simulink model "SV16"  (R2026a)
settings: Solver=VariableStepAuto  StopTime=0.1
libraries: simulink x55, hdlsllib x34
(part 1 of 2)
settings Model: Creator=Soham  LastModifiedBy=Soham

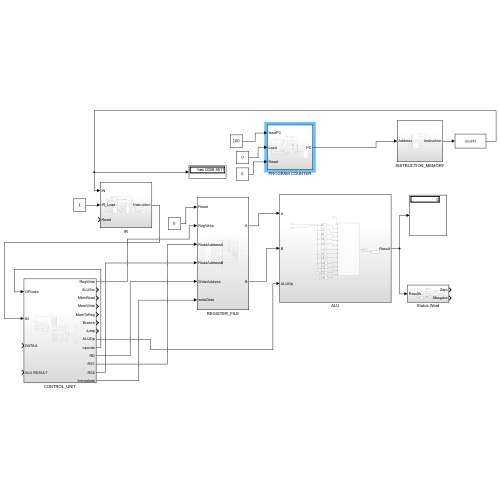
[thumbnail: Simulink's stored preview of the top-level diagram]
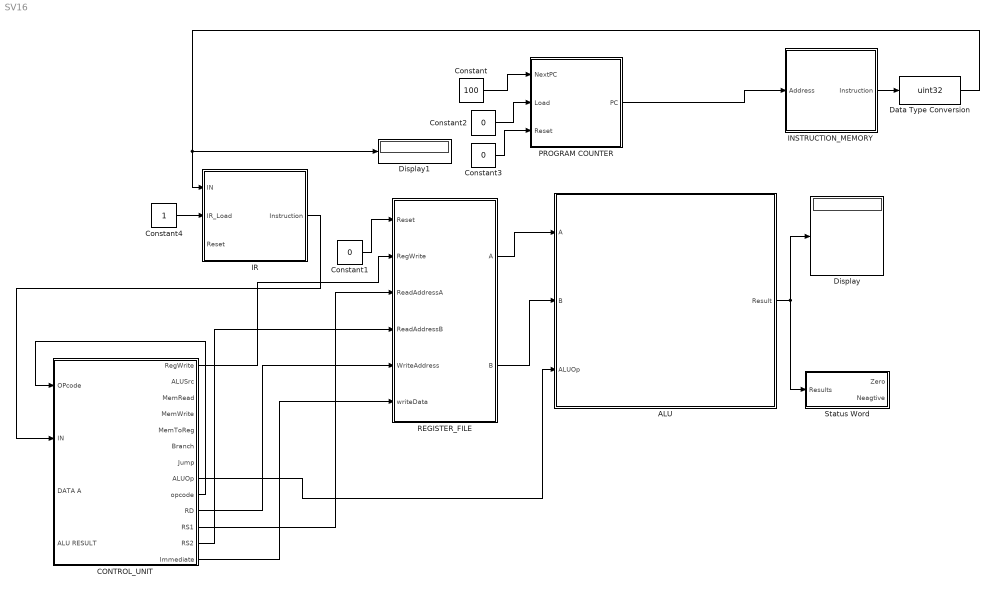
== system SV16 ==
  ALU : Subsystem
  CONTROL_UNIT : Subsystem
  Constant : Constant  Value=100  OutDataTypeStr=uint32
  Constant1 : Constant  Value=0  OutDataTypeStr=uint16
  Constant2 : Constant  Value=0  OutDataTypeStr=uint32
  Constant3 : Constant  Value=0
  Constant4 : Constant  OutDataTypeStr=uint32
  Data Type Conversion : DataTypeConversion  OutDataTypeStr=uint32  SaturateOnIntegerOverflow=off  RndMeth=Floor
  Display : Display
  Display1 : Display
      settings: Format=hex (Stored Integer)
  INSTRUCTION_MEMORY : Subsystem
  IR : Subsystem
  PROGRAM COUNTER : Subsystem
  REGISTER_FILE : Subsystem
  Status Word : Subsystem
  wires:
  Constant1/1 -> REGISTER_FILE/1(Reset)
  REGISTER_FILE/1(A) -> ALU/1(A)
  REGISTER_FILE/2(B) -> ALU/2(B)
  ALU/1(Result) -> Display/1, Status Word/1(Results)
  CONTROL_UNIT/8(ALUOp) -> ALU/3(ALUOp)
  CONTROL_UNIT/1(RegWrite) -> REGISTER_FILE/2(RegWrite)
  Data Type Conversion/1 -> IR/1(IN), Display1/1
  Constant4/1 -> IR/2(IR_Load)
  IR/1(Instruction) -> CONTROL_UNIT/2(IN)
  CONTROL_UNIT/11(RS1) -> REGISTER_FILE/3(ReadAddressA)
  CONTROL_UNIT/12(RS2) -> REGISTER_FILE/4(ReadAddressB)
  CONTROL_UNIT/10(RD) -> REGISTER_FILE/5(WriteAddress)
  CONTROL_UNIT/13(Immediate) -> REGISTER_FILE/6(writeData)
  CONTROL_UNIT/9(opcode) -> CONTROL_UNIT/1(OPcode)
  INSTRUCTION_MEMORY/1(Instruction) -> Data Type Conversion/1
  PROGRAM COUNTER/1(PC) -> INSTRUCTION_MEMORY/1(Address)
  Constant/1 -> PROGRAM COUNTER/1(NextPC)
  Constant2/1 -> PROGRAM COUNTER/2(Load)
  Constant3/1 -> PROGRAM COUNTER/3(Reset)

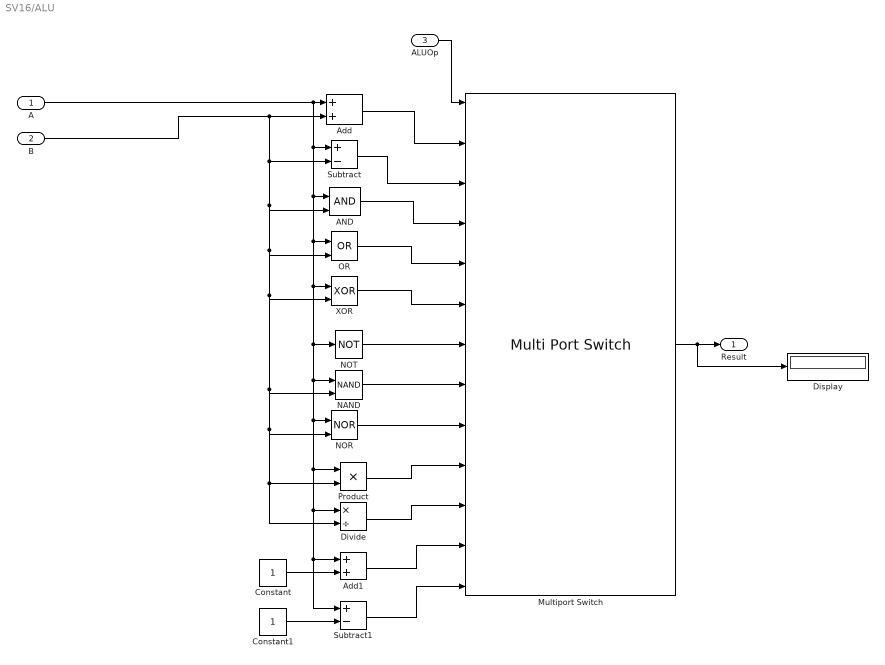
== system SV16/ALU ==
  A : Inport  OutDataTypeStr=uint16
  B : Inport  Port=2  OutDataTypeStr=uint16
  ALUOp : Inport  Port=3  OutDataTypeStr=uint8
  AND : Logic  IconShape=distinctive  AllPortsSameDT=off  OutDataTypeStr=boolean
  Add : Sum
  Add1 : Sum
  Constant : Constant  OutDataTypeStr=uint16
  Constant1 : Constant  OutDataTypeStr=uint16
  Display : Display
  Divide : Product  Inputs=*/
  Multiport Switch : MultiPortSwitch  DataPortOrder=Zero-based contiguous  Inputs=12  zeroidx=on  OutDataTypeStr=uint16  SaturateOnIntegerOverflow=off  InputSameDT=off
  NAND : Logic  Operator=NAND  IconShape=distinctive  AllPortsSameDT=off  OutDataTypeStr=boolean
  NOR : Logic  Operator=NOR  IconShape=distinctive  AllPortsSameDT=off  OutDataTypeStr=boolean
  NOT : Logic  Operator=NOT  IconShape=distinctive  AllPortsSameDT=off  OutDataTypeStr=boolean
  OR : Logic  Operator=OR  IconShape=distinctive  AllPortsSameDT=off  OutDataTypeStr=boolean
  Product : Product
  Subtract : Sum  Inputs=+-
  Subtract1 : Sum  Inputs=+-
  XOR : Logic  Operator=XOR  IconShape=distinctive  AllPortsSameDT=off  OutDataTypeStr=boolean
  Result : Outport  OutDataTypeStr=uint16
  wires:
  Constant/1 -> Add1/2
  Constant1/1 -> Subtract1/2
  ALUOp/1 -> Multiport Switch/1
  Multiport Switch/1 -> Display/1, Result/1
  A/1 -> AND/1, Subtract1/1, Add1/1, Divide/1, Product/1, NOR/1, NAND/1, NOT/1, XOR/1, OR/1, Subtract/1, Add/1
  Add/1 -> Multiport Switch/2
  Subtract/1 -> Multiport Switch/3
  AND/1 -> Multiport Switch/4
  OR/1 -> Multiport Switch/5
  XOR/1 -> Multiport Switch/6
  NOT/1 -> Multiport Switch/7
  NAND/1 -> Multiport Switch/8
  NOR/1 -> Multiport Switch/9
  Subtract1/1 -> Multiport Switch/13
  Add1/1 -> Multiport Switch/12
  Divide/1 -> Multiport Switch/11
  Product/1 -> Multiport Switch/10
  B/1 -> NAND/2, Divide/2, Product/2, NOR/2, XOR/2, OR/2, AND/2, Subtract/2, Add/2

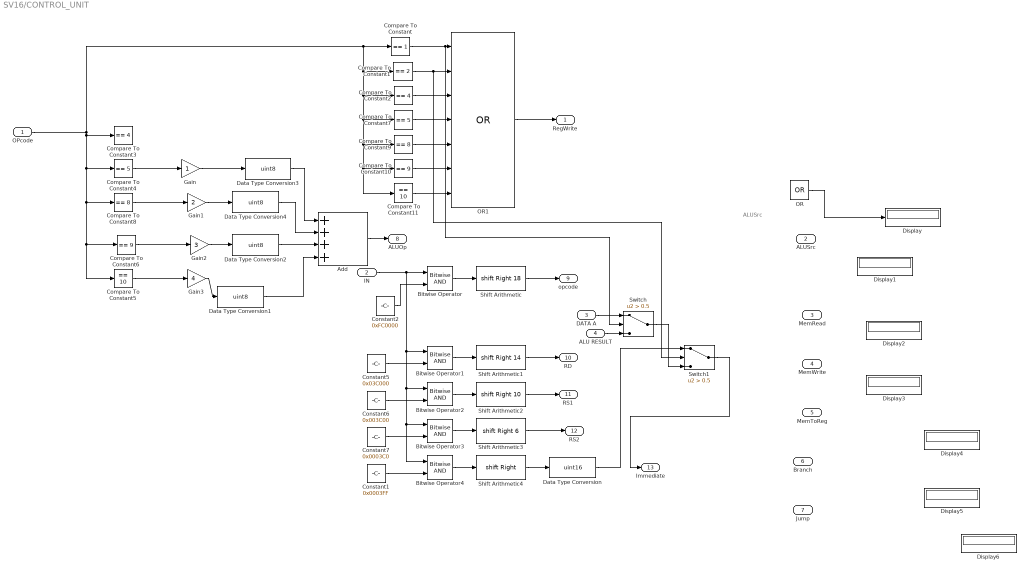
== system SV16/CONTROL_UNIT ==
  note: ALUSrc
  OPcode : Inport  OutDataTypeStr=uint32  PortDimensions=1
  IN : Inport  Port=2
  DATA A : Inport  Port=3
  ALU RESULT : Inport  Port=4
  Add : Sum  Inputs=++++
  Bitwise Operator{,1..4} (5 alike) : simulink/Logic and Bit Operations/Bitwise Operator  logicop=AND  UseBitMask=off  NumInputPorts=2  BitMask=bin2dec('11011001')  BitMaskRealWorld=Stored Integer
  Compare To Constant : simulink/Logic and Bit Operations/Compare To Constant  relop===  const=1  OutDataTypeStr=boolean
  Compare To Constant1 : simulink/Logic and Bit Operations/Compare To Constant  relop===  const=2  OutDataTypeStr=boolean
  Compare To Constant10 : simulink/Logic and Bit Operations/Compare To Constant  relop===  const=9  OutDataTypeStr=boolean
  Compare To Constant11 : simulink/Logic and Bit Operations/Compare To Constant  relop===  const=10  OutDataTypeStr=boolean
  Compare To Constant2 : simulink/Logic and Bit Operations/Compare To Constant  relop===  const=4  OutDataTypeStr=boolean
  Compare To Constant3 : simulink/Logic and Bit Operations/Compare To Constant  relop===  const=4  OutDataTypeStr=boolean
  Compare To Constant4 : simulink/Logic and Bit Operations/Compare To Constant  relop===  const=5  OutDataTypeStr=boolean
  Compare To Constant5 : simulink/Logic and Bit Operations/Compare To Constant  relop===  const=10  OutDataTypeStr=boolean
  Compare To Constant6 : simulink/Logic and Bit Operations/Compare To Constant  relop===  const=9  OutDataTypeStr=boolean
  Compare To Constant7 : simulink/Logic and Bit Operations/Compare To Constant  relop===  const=5  OutDataTypeStr=boolean
  Compare To Constant8 : simulink/Logic and Bit Operations/Compare To Constant  relop===  const=8  OutDataTypeStr=boolean
  Compare To Constant9 : simulink/Logic and Bit Operations/Compare To Constant  relop===  const=8  OutDataTypeStr=boolean
  Constant1 : Constant  Value=0x0003FF
  Constant2 : Constant  Value=0xFC0000
  Constant5 : Constant  Value=0x03C000
  Constant6 : Constant  Value=0x003C00
  Constant7 : Constant  Value=0x0003C0
  Data Type Conversion : DataTypeConversion  OutDataTypeStr=uint16  SaturateOnIntegerOverflow=off  RndMeth=Floor
  Data Type Conversion{1..4} (4 alike) : DataTypeConversion  OutDataTypeStr=uint8  SaturateOnIntegerOverflow=off  RndMeth=Floor
  Display{,1..6} (7 alike) : Display
  Gain : Gain
  Gain1 : Gain  Gain=2
  Gain2 : Gain  Gain=3
  Gain3 : Gain  Gain=4
  OR : Logic  Operator=OR  IconShape=distinctive  AllPortsSameDT=off  OutDataTypeStr=boolean
  OR1 : Logic  Operator=OR  Inputs=7  IconShape=distinctive  AllPortsSameDT=off  OutDataTypeStr=boolean
  Shift Arithmetic : ArithShift  BitShiftNumber=18  BitShiftDirection=Right
  Shift Arithmetic1 : ArithShift  BitShiftNumber=14  BitShiftDirection=Right
  Shift Arithmetic2 : ArithShift  BitShiftNumber=10  BitShiftDirection=Right
  Shift Arithmetic3 : ArithShift  BitShiftNumber=6  BitShiftDirection=Right
  Shift Arithmetic4 : ArithShift  BitShiftDirection=Right
  Switch : Switch  Criteria=u2 > Threshold  Threshold=0.5  SaturateOnIntegerOverflow=off  InputSameDT=off
  Switch1 : Switch  Criteria=u2 > Threshold  Threshold=0.5  SaturateOnIntegerOverflow=off  InputSameDT=off
  RegWrite : Outport  OutDataTypeStr=boolean
  ALUSrc : Outport  Port=2  OutDataTypeStr=boolean
  MemRead : Outport  Port=3  OutDataTypeStr=boolean
  MemWrite : Outport  Port=4  OutDataTypeStr=boolean
  MemToReg : Outport  Port=5  OutDataTypeStr=boolean
  Branch : Outport  Port=6  OutDataTypeStr=boolean
  Jump : Outport  Port=7  OutDataTypeStr=boolean
  ALUOp : Outport  Port=8  OutDataTypeStr=uint8
  opcode : Outport  Port=9
  RD : Outport  Port=10
  RS1 : Outport  Port=11
  RS2 : Outport  Port=12
  Immediate : Outport  Port=13
  wires:
  ? -> OR/1
  ? -> OR/2
  OR/1 -> Display/1
  ? -> Display1/1, ALUSrc/1
  ? -> Display2/1, MemRead/1
  ? -> Display3/1, MemWrite/1
  ? -> Display4/1, MemToReg/1
  ? -> Display5/1, Branch/1
  ? -> Display6/1, Jump/1
  OPcode/1 -> Compare To Constant11/1, Compare To Constant10/1, Compare To Constant9/1, Compare To Constant7/1, Compare To Constant2/1, Compare To Constant1/1, Compare To Constant/1, Compare To Constant4/1, Compare To Constant5/1, Compare To Constant6/1, Compare To Constant8/1, Compare To Constant3/1
  Compare To Constant/1 -> OR1/1, Switch/2
  Compare To Constant8/1 -> Gain1/1
  Compare To Constant4/1 -> Gain/1
  Compare To Constant6/1 -> Gain2/1
  Compare To Constant5/1 -> Gain3/1
  Compare To Constant1/1 -> Switch1/2, OR1/2
  Gain/1 -> Data Type Conversion3/1
  Gain2/1 -> Data Type Conversion2/1
  Gain1/1 -> Data Type Conversion4/1
  Gain3/1 -> Data Type Conversion1/1
  Add/1 -> ALUOp/1
  Compare To Constant2/1 -> OR1/3
  Compare To Constant7/1 -> OR1/4
  Compare To Constant9/1 -> OR1/5
  Compare To Constant10/1 -> OR1/6
  Compare To Constant11/1 -> OR1/7
  OR1/1 -> RegWrite/1
  Bitwise Operator3/1 -> Shift Arithmetic3/1
  Constant7/1 -> Bitwise Operator3/2
  Bitwise Operator2/1 -> Shift Arithmetic2/1
  Constant2/1 -> Bitwise Operator/2
  Bitwise Operator/1 -> Shift Arithmetic/1
  Constant5/1 -> Bitwise Operator1/2
  Bitwise Operator1/1 -> Shift Arithmetic1/1
  Constant1/1 -> Bitwise Operator4/2
  Shift Arithmetic1/1 -> RD/1
  Shift Arithmetic3/1 -> RS2/1
  Constant6/1 -> Bitwise Operator2/2
  Bitwise Operator4/1 -> Shift Arithmetic4/1
  Shift Arithmetic4/1 -> Data Type Conversion/1
  Shift Arithmetic/1 -> opcode/1
  Shift Arithmetic2/1 -> RS1/1
  IN/1 -> Bitwise Operator4/1, Bitwise Operator3/1, Bitwise Operator2/1, Bitwise Operator1/1, Bitwise Operator/1
  DATA A/1 -> Switch/1
  ALU RESULT/1 -> Switch/3
  Switch/1 -> Switch1/3
  Data Type Conversion/1 -> Switch1/1
  Switch1/1 -> Immediate/1
  Data Type Conversion1/1 -> Add/4
  Data Type Conversion2/1 -> Add/3
  Data Type Conversion3/1 -> Add/1
  Data Type Conversion4/1 -> Add/2

== system SV16/INSTRUCTION_MEMORY ==
  Address : Inport  OutDataTypeStr=uint32
  Compare To Constant : simulink/Logic and Bit Operations/Compare To Constant  relop=>=  const=8  OutDataTypeStr=boolean
  Constant : Constant  Value=0x088011  VectorParams1D=off
  Constant1 : Constant  OutDataTypeStr=boolean
  Constant2 : Constant  Value=0x088011  VectorParams1D=off
  Data Type Conversion : DataTypeConversion  OutDataTypeStr=uint32  SaturateOnIntegerOverflow=off  RndMeth=Floor
  Display : Display
      settings: Format=hex (Stored Integer)
  Display1 : Display
      settings: Format=hex (Stored Integer)
  Display2 : Display
      settings: Format=hex (Stored Integer)
  MEMORY_BANK_8_B0 : Subsystem
  MEMORY_BANK_8_B1 : Subsystem
  Subsystem : Subsystem
  Switch : Switch  Criteria=u2 ~= 0  SaturateOnIntegerOverflow=off  InputSameDT=off
  Instruction : Outport  OutDataTypeStr=uint32
  wires:
  MEMORY_BANK_8_B0/1(DataOut) -> Switch/3, Display/1
  Address/1 -> Subsystem/1(IN)
  Subsystem/1(AD0) -> MEMORY_BANK_8_B0/2(Address0)
  Subsystem/2(AD1) -> MEMORY_BANK_8_B0/3(Address1)
  Subsystem/3(AD2) -> MEMORY_BANK_8_B0/4(Address2)
  Subsystem/4(INSTRUCTION INDEX) -> Compare To Constant/1
  Compare To Constant/1 -> Switch/2
  MEMORY_BANK_8_B1/1(DataOut) -> Switch/1, Display1/1
  Switch/1 -> Display2/1, Data Type Conversion/1
  Data Type Conversion/1 -> Instruction/1
  Constant/1 -> MEMORY_BANK_8_B0/1(DataIn)
  Constant1/1 -> MEMORY_BANK_8_B0/6(WriteEnable), MEMORY_BANK_8_B1/6(WriteEnable)
  Constant2/1 -> MEMORY_BANK_8_B1/1(DataIn)

== system SV16/IR ==
  IN : Inport  OutDataTypeStr=uint32
  IR_Load : Inport  Port=2  OutDataTypeStr=uint32
  Reset : Inport  Port=3  OutDataTypeStr=uint32
  Constant : Constant  Value=0  OutDataTypeStr=uint32
  Constant1 : Constant  OutDataTypeStr=uint32
  Display : Display
  Switch : Switch  Criteria=u2 > Threshold  SaturateOnIntegerOverflow=off  InputSameDT=off
  Switch1 : Switch  Criteria=u2 > Threshold  OutDataTypeStr=uint32  SaturateOnIntegerOverflow=off  InputSameDT=off
  Unit Delay Enabled Synchronous : hdlsllib/Discrete/Unit Delay Enabled Synchronous  InitialCondition=0.0  SampleTime=-1
  Instruction : Outport  OutDataTypeStr=uint32  PortDimensions=1
  wires:
  IN/1 -> Switch/1
  IR_Load/1 -> Switch/2
  Reset/1 -> Switch1/2
  Constant/1 -> Switch1/1
  Switch/1 -> Switch1/3
  Unit Delay Enabled Synchronous/1 -> Switch/3, Display/1, Instruction/1
  Switch1/1 -> Unit Delay Enabled Synchronous/1
  Constant1/1 -> Unit Delay Enabled Synchronous/2

== system SV16/PROGRAM COUNTER ==
  NextPC : Inport  OutDataTypeStr=uint32
  Load : Inport  Port=2  OutDataTypeStr=uint32
  Reset : Inport  Port=3
  Add : Sum
  Constant1 : Constant
  Constant2 : Constant  Value=3
  Constant3 : Constant  Value=0
  Data Type Conversion : DataTypeConversion  OutDataTypeStr=uint32  SaturateOnIntegerOverflow=off  RndMeth=Floor
  Data Type Conversion1 : DataTypeConversion  OutDataTypeStr=uint32  SaturateOnIntegerOverflow=off  RndMeth=Floor
  Display : Display
      settings: Format=decimal (Stored Integer)
  Unit Delay Enabled Synchronous : hdlsllib/Discrete/Unit Delay Enabled Synchronous  InitialCondition=0.0  SampleTime=0.001
  pc switch : Switch  Criteria=u2 > Threshold  OutDataTypeStr=uint32  SaturateOnIntegerOverflow=off  InputSameDT=off
  reset switch : Switch  Criteria=u2 > Threshold  SaturateOnIntegerOverflow=off  InputSameDT=off
  PC : Outport  OutDataTypeStr=uint32
  wires:
  Constant1/1 -> Unit Delay Enabled Synchronous/2
  Unit Delay Enabled Synchronous/1 -> Add/2, PC/1, Display/1
  Constant2/1 -> Add/1
  NextPC/1 -> pc switch/1
  Load/1 -> pc switch/2
  Add/1 -> pc switch/3
  Constant3/1 -> reset switch/1
  Reset/1 -> reset switch/2
  pc switch/1 -> Data Type Conversion1/1
  reset switch/1 -> Data Type Conversion/1
  Data Type Conversion/1 -> Unit Delay Enabled Synchronous/1
  Data Type Conversion1/1 -> reset switch/3

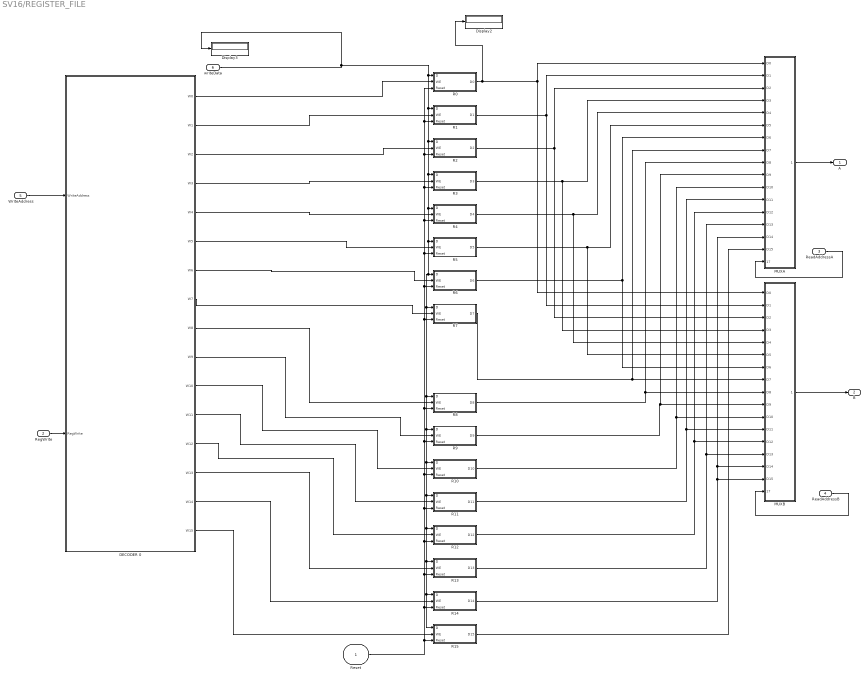
== system SV16/REGISTER_FILE ==
  Reset : Inport
  RegWrite : Inport  Port=2
  ReadAddressA : Inport  Port=3
  ReadAddressB : Inport  Port=4
  WriteAddress : Inport  Port=5
  writeData : Inport  Port=6
  DECODER 0 : Subsystem
  Display2 : Display
  Display3 : Display
  MUXA : Subsystem
  MUXB : Subsystem
  R0 : Subsystem
  R1 : Subsystem
  R10 : Subsystem
  R11 : Subsystem
  R12 : Subsystem
  R13 : Subsystem
  R14 : Subsystem
  R15 : Subsystem
  R2 : Subsystem
  R3 : Subsystem
  R4 : Subsystem
  R5 : Subsystem
  R6 : Subsystem
  R7 : Subsystem
  R8 : Subsystem
  R9 : Subsystem
  A : Outport  OutDataTypeStr=uint16
  B : Outport  Port=2  OutDataTypeStr=uint16
  wires:
  DECODER 0/1(W0) -> R0/2(WE)
  DECODER 0/2(W1) -> R1/2(WE)
  DECODER 0/3(W2) -> R2/2(WE)
  DECODER 0/4(W3) -> R3/2(WE)
  DECODER 0/5(W4) -> R4/2(WE)
  DECODER 0/6(W5) -> R5/2(WE)
  DECODER 0/7(W6) -> R6/2(WE)
  DECODER 0/8(W7) -> R7/2(WE)
  R0/1(D0) -> Display2/1, MUXA/1(D0), MUXB/1(D0)
  R1/1(D1) -> MUXA/2(D1), MUXB/2(D1)
  R2/1(D2) -> MUXB/3(D2), MUXA/3(D2)
  R3/1(D3) -> MUXA/4(D3), MUXB/4(D3)
  R4/1(D4) -> MUXB/5(D4), MUXA/5(D4)
  R5/1(D5) -> MUXB/6(D5), MUXA/6(D5)
  R6/1(D6) -> MUXB/7(D6), MUXA/7(D6)
  R7/1(D7) -> MUXA/8(D7), MUXB/8(D7)
  writeData/1 -> R1/1(D), R2/1(D), R3/1(D), R4/1(D), R5/1(D), R15/1(D), R14/1(D), R13/1(D), R12/1(D), R11/1(D), R10/1(D), R9/1(D), R8/1(D), R7/1(D), R6/1(D), R0/1(D), Display3/1
  Reset/1 -> R13/3(Reset), R12/3(Reset), R11/3(Reset), R9/3(Reset), R8/3(Reset), R7/3(Reset), R6/3(Reset), R5/3(Reset), R4/3(Reset), R3/3(Reset), R2/3(Reset), R1/3(Reset), R0/3(Reset), R10/3(Reset), R14/3(Reset), R15/3(Reset)
  WriteAddress/1 -> DECODER 0/1(WriteAddress)
  RegWrite/1 -> DECODER 0/2(RegWrite)
  MUXA/1(ReadDataA) -> A/1
  MUXB/1(ReadDataB) -> B/1
  ReadAddressA/1 -> MUXA/17(ReadAddressA)
  ReadAddressB/1 -> MUXB/17(ReadAddressB)
  DECODER 0/9(W8) -> R8/2(WE)
  DECODER 0/10(W9) -> R9/2(WE)
  DECODER 0/11(W10) -> R10/2(WE)
  DECODER 0/12(W11) -> R11/2(WE)
  DECODER 0/13(W12) -> R12/2(WE)
  DECODER 0/14(W13) -> R13/2(WE)
  DECODER 0/15(W14) -> R14/2(WE)
  DECODER 0/16(W15) -> R15/2(WE)
  R8/1(D8) -> MUXA/9(D8), MUXB/9(D8)
  R9/1(D9) -> MUXA/10(D9), MUXB/10(D9)
  R10/1(D10) -> MUXA/11(D10), MUXB/11(D10)
  R11/1(D11) -> MUXA/12(D11), MUXB/12(D11)
  R12/1(D12) -> MUXA/13(D12), MUXB/13(D12)
  R13/1(D13) -> MUXA/14(D13), MUXB/14(D13)
  R14/1(D14) -> MUXA/15(D14), MUXB/15(D14), MUXB/16(D15)
  R15/1(D15) -> MUXA/16(D15)

== system SV16/Status Word ==
  Results : Inport  OutDataTypeStr=uint16
  Compare To Constant : simulink/Logic and Bit Operations/Compare To Constant  relop===  const=0  OutDataTypeStr=boolean
  Compare To Constant1 : simulink/Logic and Bit Operations/Compare To Constant  relop=>=  const=32768  OutDataTypeStr=boolean
  Display : Display
  Display1 : Display
  Zero : Outport  OutDataTypeStr=boolean
  Neagtive : Outport  Port=2
  wires:
  Results/1 -> Compare To Constant/1, Compare To Constant1/1
  Compare To Constant/1 -> Display/1, Zero/1
  Compare To Constant1/1 -> Display1/1, Neagtive/1

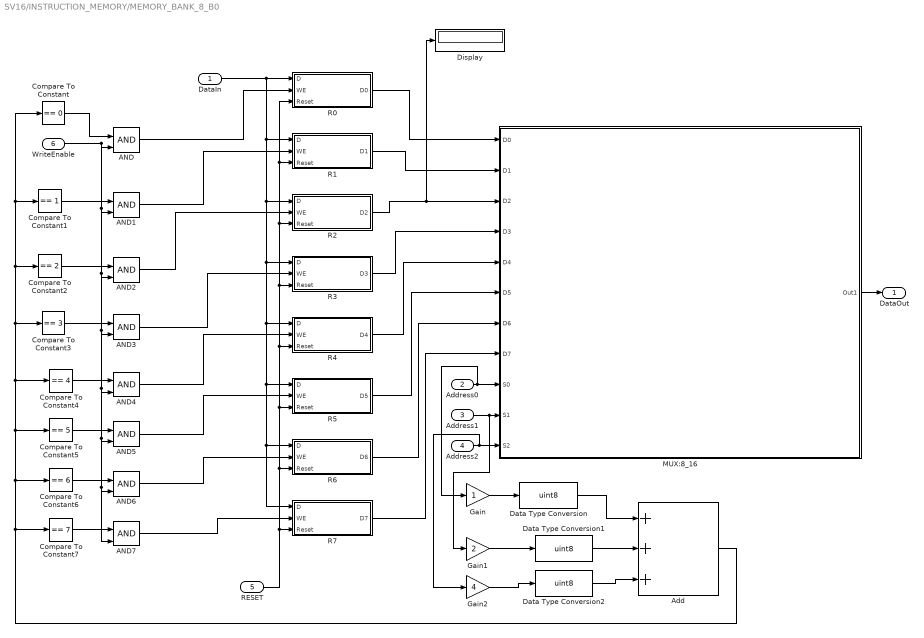
== system SV16/INSTRUCTION_MEMORY/MEMORY_BANK_8_B0 ==
  DataIn : Inport  OutDataTypeStr=uint32
  Address0 : Inport  Port=2  OutDataTypeStr=boolean
  Address1 : Inport  Port=3  OutDataTypeStr=boolean
  Address2 : Inport  Port=4  OutDataTypeStr=boolean
  RESET : Inport  Port=5  OutDataTypeStr=boolean
  WriteEnable : Inport  Port=6  OutDataTypeStr=boolean
  AND{,1..7} (8 alike) : Logic  IconShape=distinctive  AllPortsSameDT=off  OutDataTypeStr=boolean
  Add : Sum  Inputs=+++  OutDataTypeStr=Inherit: Inherit via back propagation
  Compare To Constant : simulink/Logic and Bit Operations/Compare To Constant  relop===  const=0  OutDataTypeStr=boolean
  Compare To Constant1 : simulink/Logic and Bit Operations/Compare To Constant  relop===  const=1  OutDataTypeStr=boolean
  Compare To Constant2 : simulink/Logic and Bit Operations/Compare To Constant  relop===  const=2  OutDataTypeStr=boolean
  Compare To Constant3 : simulink/Logic and Bit Operations/Compare To Constant  relop===  const=3  OutDataTypeStr=boolean
  Compare To Constant4 : simulink/Logic and Bit Operations/Compare To Constant  relop===  const=4  OutDataTypeStr=boolean
  Compare To Constant5 : simulink/Logic and Bit Operations/Compare To Constant  relop===  const=5  OutDataTypeStr=boolean
  Compare To Constant6 : simulink/Logic and Bit Operations/Compare To Constant  relop===  const=6  OutDataTypeStr=boolean
  Compare To Constant7 : simulink/Logic and Bit Operations/Compare To Constant  relop===  const=7  OutDataTypeStr=boolean
  Data Type Conversion : DataTypeConversion  OutDataTypeStr=uint8  SaturateOnIntegerOverflow=off  RndMeth=Floor
  Data Type Conversion1 : DataTypeConversion  OutDataTypeStr=uint8  SaturateOnIntegerOverflow=off  RndMeth=Floor
  Data Type Conversion2 : DataTypeConversion  OutDataTypeStr=uint8  SaturateOnIntegerOverflow=off  RndMeth=Floor
  Display : Display
  Gain : Gain
  Gain1 : Gain  Gain=2
  Gain2 : Gain  Gain=4
  MUX:8_16 : Subsystem
  R0 : Subsystem
  R1 : Subsystem
  R2 : Subsystem
  R3 : Subsystem
  R4 : Subsystem
  R5 : Subsystem
  R6 : Subsystem
  R7 : Subsystem
  DataOut : Outport  OutDataTypeStr=uint32
  wires:
  DataIn/1 -> R4/1(D), R7/1(D), R6/1(D), R5/1(D), R3/1(D), R2/1(D), R1/1(D), R0/1(D)
  Address0/1 -> Gain/1, MUX:8_16/9(S0)
  Address1/1 -> Gain1/1, MUX:8_16/10(S1)
  Address2/1 -> Gain2/1, MUX:8_16/11(S2)
  R0/1(D0) -> MUX:8_16/1(D0)
  R2/1(D2) -> Display/1, MUX:8_16/3(D2)
  R1/1(D1) -> MUX:8_16/2(D1)
  R3/1(D3) -> MUX:8_16/4(D3)
  R4/1(D4) -> MUX:8_16/5(D4)
  R5/1(D5) -> MUX:8_16/6(D5)
  R6/1(D6) -> MUX:8_16/7(D6)
  R7/1(D7) -> MUX:8_16/8(D7)
  MUX:8_16/1(Out1) -> DataOut/1
  AND/1 -> R0/2(WE)
  Gain/1 -> Data Type Conversion/1
  Gain1/1 -> Data Type Conversion1/1
  Gain2/1 -> Data Type Conversion2/1
  Add/1 -> Compare To Constant7/1, Compare To Constant6/1, Compare To Constant/1, Compare To Constant1/1, Compare To Constant2/1, Compare To Constant3/1, Compare To Constant4/1, Compare To Constant5/1
  Compare To Constant/1 -> AND/1
  Compare To Constant1/1 -> AND1/1
  Compare To Constant3/1 -> AND3/1
  WriteEnable/1 -> AND7/2, AND6/2, AND5/2, AND4/2, AND3/2, AND2/2, AND1/2, AND/2
  Compare To Constant2/1 -> AND2/1
  Compare To Constant7/1 -> AND7/1
  Compare To Constant6/1 -> AND6/1
  Compare To Constant5/1 -> AND5/1
  Compare To Constant4/1 -> AND4/1
  AND1/1 -> R1/2(WE)
  AND2/1 -> R2/2(WE)
  AND4/1 -> R4/2(WE)
  AND3/1 -> R3/2(WE)
  AND5/1 -> R5/2(WE)
  AND6/1 -> R6/2(WE)
  AND7/1 -> R7/2(WE)
  RESET/1 -> R0/3(Reset), R1/3(Reset), R2/3(Reset), R3/3(Reset), R4/3(Reset), R5/3(Reset), R6/3(Reset), R7/3(Reset)
  Data Type Conversion/1 -> Add/1
  Data Type Conversion1/1 -> Add/2
  Data Type Conversion2/1 -> Add/3

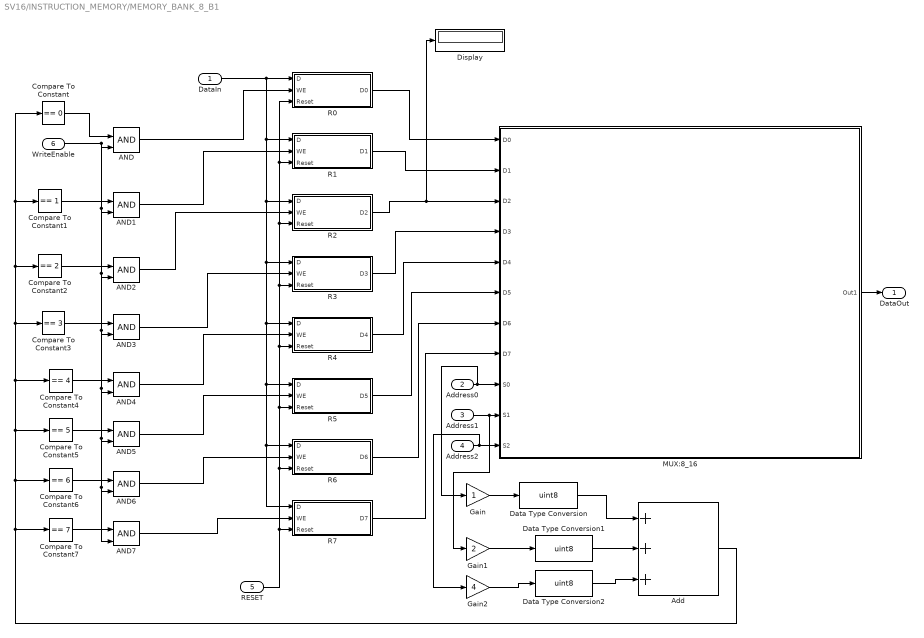
== system SV16/INSTRUCTION_MEMORY/MEMORY_BANK_8_B1 ==
  DataIn : Inport  OutDataTypeStr=uint32
  Address0 : Inport  Port=2  OutDataTypeStr=boolean
  Address1 : Inport  Port=3  OutDataTypeStr=boolean
  Address2 : Inport  Port=4  OutDataTypeStr=boolean
  RESET : Inport  Port=5  OutDataTypeStr=boolean
  WriteEnable : Inport  Port=6  OutDataTypeStr=boolean
  AND{,1..7} (8 alike) : Logic  IconShape=distinctive  AllPortsSameDT=off  OutDataTypeStr=boolean
  Add : Sum  Inputs=+++  OutDataTypeStr=Inherit: Inherit via back propagation
  Compare To Constant : simulink/Logic and Bit Operations/Compare To Constant  relop===  const=0  OutDataTypeStr=boolean
  Compare To Constant1 : simulink/Logic and Bit Operations/Compare To Constant  relop===  const=1  OutDataTypeStr=boolean
  Compare To Constant2 : simulink/Logic and Bit Operations/Compare To Constant  relop===  const=2  OutDataTypeStr=boolean
  Compare To Constant3 : simulink/Logic and Bit Operations/Compare To Constant  relop===  const=3  OutDataTypeStr=boolean
  Compare To Constant4 : simulink/Logic and Bit Operations/Compare To Constant  relop===  const=4  OutDataTypeStr=boolean
  Compare To Constant5 : simulink/Logic and Bit Operations/Compare To Constant  relop===  const=5  OutDataTypeStr=boolean
  Compare To Constant6 : simulink/Logic and Bit Operations/Compare To Constant  relop===  const=6  OutDataTypeStr=boolean
  Compare To Constant7 : simulink/Logic and Bit Operations/Compare To Constant  relop===  const=7  OutDataTypeStr=boolean
  Data Type Conversion : DataTypeConversion  OutDataTypeStr=uint8  SaturateOnIntegerOverflow=off  RndMeth=Floor
  Data Type Conversion1 : DataTypeConversion  OutDataTypeStr=uint8  SaturateOnIntegerOverflow=off  RndMeth=Floor
  Data Type Conversion2 : DataTypeConversion  OutDataTypeStr=uint8  SaturateOnIntegerOverflow=off  RndMeth=Floor
  Display : Display
  Gain : Gain
  Gain1 : Gain  Gain=2
  Gain2 : Gain  Gain=4
  MUX:8_16 : Subsystem
  R0 : Subsystem
  R1 : Subsystem
  R2 : Subsystem
  R3 : Subsystem
  R4 : Subsystem
  R5 : Subsystem
  R6 : Subsystem
  R7 : Subsystem
  DataOut : Outport  OutDataTypeStr=uint32
  wires:
  DataIn/1 -> R4/1(D), R7/1(D), R6/1(D), R5/1(D), R3/1(D), R2/1(D), R1/1(D), R0/1(D)
  Address0/1 -> Gain/1, MUX:8_16/9(S0)
  Address1/1 -> Gain1/1, MUX:8_16/10(S1)
  Address2/1 -> Gain2/1, MUX:8_16/11(S2)
  R0/1(D0) -> MUX:8_16/1(D0)
  R2/1(D2) -> Display/1, MUX:8_16/3(D2)
  R1/1(D1) -> MUX:8_16/2(D1)
  R3/1(D3) -> MUX:8_16/4(D3)
  R4/1(D4) -> MUX:8_16/5(D4)
  R5/1(D5) -> MUX:8_16/6(D5)
  R6/1(D6) -> MUX:8_16/7(D6)
  R7/1(D7) -> MUX:8_16/8(D7)
  MUX:8_16/1(Out1) -> DataOut/1
  AND/1 -> R0/2(WE)
  Gain/1 -> Data Type Conversion/1
  Gain1/1 -> Data Type Conversion1/1
  Gain2/1 -> Data Type Conversion2/1
  Add/1 -> Compare To Constant7/1, Compare To Constant6/1, Compare To Constant/1, Compare To Constant1/1, Compare To Constant2/1, Compare To Constant3/1, Compare To Constant4/1, Compare To Constant5/1
  Compare To Constant/1 -> AND/1
  Compare To Constant1/1 -> AND1/1
  Compare To Constant3/1 -> AND3/1
  WriteEnable/1 -> AND7/2, AND6/2, AND5/2, AND4/2, AND3/2, AND2/2, AND1/2, AND/2
  Compare To Constant2/1 -> AND2/1
  Compare To Constant7/1 -> AND7/1
  Compare To Constant6/1 -> AND6/1
  Compare To Constant5/1 -> AND5/1
  Compare To Constant4/1 -> AND4/1
  AND1/1 -> R1/2(WE)
  AND2/1 -> R2/2(WE)
  AND4/1 -> R4/2(WE)
  AND3/1 -> R3/2(WE)
  AND5/1 -> R5/2(WE)
  AND6/1 -> R6/2(WE)
  AND7/1 -> R7/2(WE)
  RESET/1 -> R0/3(Reset), R1/3(Reset), R2/3(Reset), R3/3(Reset), R4/3(Reset), R5/3(Reset), R6/3(Reset), R7/3(Reset)
  Data Type Conversion/1 -> Add/1
  Data Type Conversion1/1 -> Add/2
  Data Type Conversion2/1 -> Add/3

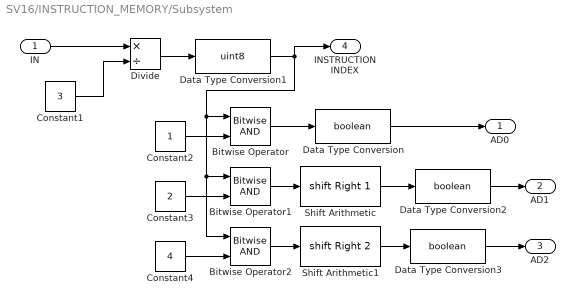
== system SV16/INSTRUCTION_MEMORY/Subsystem ==
  IN : Inport
  Bitwise Operator : simulink/Logic and Bit Operations/Bitwise Operator  logicop=AND  UseBitMask=off  NumInputPorts=2  BitMask=bin2dec('11011001')  BitMaskRealWorld=Stored Integer
  Bitwise Operator1 : simulink/Logic and Bit Operations/Bitwise Operator  logicop=AND  UseBitMask=off  NumInputPorts=2  BitMask=bin2dec('11011001')  BitMaskRealWorld=Stored Integer
  Bitwise Operator2 : simulink/Logic and Bit Operations/Bitwise Operator  logicop=AND  UseBitMask=off  NumInputPorts=2  BitMask=bin2dec('11011001')  BitMaskRealWorld=Stored Integer
  Constant1 : Constant  Value=3  OutDataTypeStr=uint32
  Constant2 : Constant  OutDataTypeStr=uint8
  Constant3 : Constant  Value=2  OutDataTypeStr=uint8
  Constant4 : Constant  Value=4  OutDataTypeStr=uint8
  Data Type Conversion : DataTypeConversion  OutDataTypeStr=boolean  SaturateOnIntegerOverflow=off  RndMeth=Floor
  Data Type Conversion1 : DataTypeConversion  OutDataTypeStr=uint8  SaturateOnIntegerOverflow=off  RndMeth=Floor
  Data Type Conversion2 : DataTypeConversion  OutDataTypeStr=boolean  SaturateOnIntegerOverflow=off  RndMeth=Floor
  Data Type Conversion3 : DataTypeConversion  OutDataTypeStr=boolean  SaturateOnIntegerOverflow=off  RndMeth=Floor
  Divide : Product  Inputs=*/
  Shift Arithmetic : ArithShift  BitShiftNumber=1  BitShiftDirection=Right
  Shift Arithmetic1 : ArithShift  BitShiftNumber=2  BitShiftDirection=Right
  AD0 : Outport
  AD1 : Outport  Port=2
  AD2 : Outport  Port=3
  INSTRUCTION INDEX : Outport  Port=4
  wires:
  Constant3/1 -> Bitwise Operator1/2
  Divide/1 -> Data Type Conversion1/1
  Data Type Conversion1/1 -> INSTRUCTION INDEX/1, Bitwise Operator2/1, Bitwise Operator1/1, Bitwise Operator/1
  Bitwise Operator2/1 -> Shift Arithmetic1/1
  Constant2/1 -> Bitwise Operator/2
  IN/1 -> Divide/1
  Constant4/1 -> Bitwise Operator2/2
  Constant1/1 -> Divide/2
  Bitwise Operator1/1 -> Shift Arithmetic/1
  Shift Arithmetic1/1 -> Data Type Conversion3/1
  Shift Arithmetic/1 -> Data Type Conversion2/1
  Bitwise Operator/1 -> Data Type Conversion/1
  Data Type Conversion/1 -> AD0/1
  Data Type Conversion2/1 -> AD1/1
  Data Type Conversion3/1 -> AD2/1

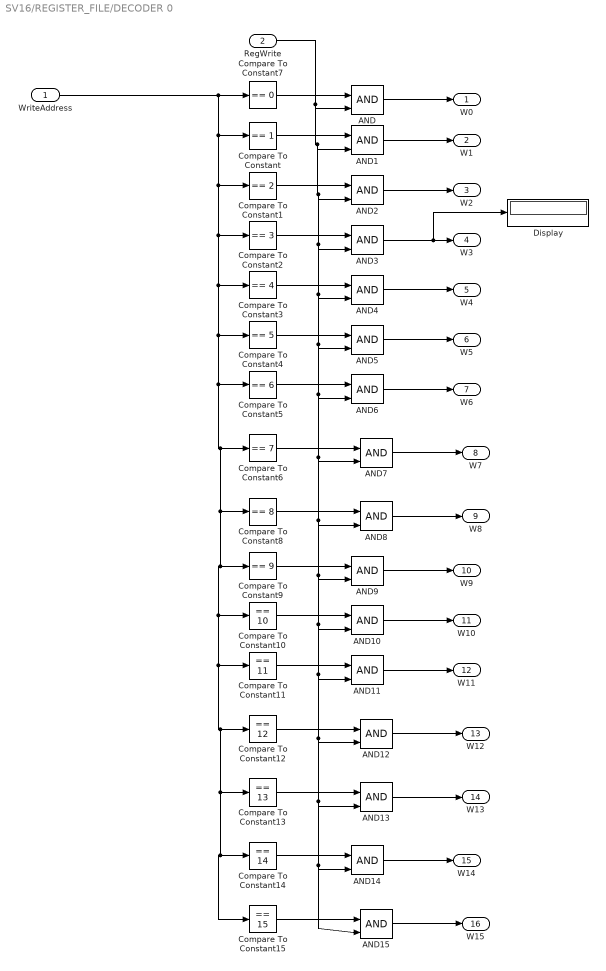
== system SV16/REGISTER_FILE/DECODER 0 ==
  WriteAddress : Inport  PortDimensions=1
  RegWrite : Inport  Port=2
  AND{,1..15} (16 alike) : Logic  IconShape=distinctive  AllPortsSameDT=off  OutDataTypeStr=boolean
  Compare To Constant : simulink/Logic and Bit Operations/Compare To Constant  relop===  const=1  OutDataTypeStr=boolean
  Compare To Constant1 : simulink/Logic and Bit Operations/Compare To Constant  relop===  const=2  OutDataTypeStr=boolean
  Compare To Constant10 : simulink/Logic and Bit Operations/Compare To Constant  relop===  const=10  OutDataTypeStr=boolean
  Compare To Constant11 : simulink/Logic and Bit Operations/Compare To Constant  relop===  const=11  OutDataTypeStr=boolean
  Compare To Constant12 : simulink/Logic and Bit Operations/Compare To Constant  relop===  const=12  OutDataTypeStr=boolean
  Compare To Constant13 : simulink/Logic and Bit Operations/Compare To Constant  relop===  const=13  OutDataTypeStr=boolean
  Compare To Constant14 : simulink/Logic and Bit Operations/Compare To Constant  relop===  const=14  OutDataTypeStr=boolean
  Compare To Constant15 : simulink/Logic and Bit Operations/Compare To Constant  relop===  const=15  OutDataTypeStr=boolean
  Compare To Constant2 : simulink/Logic and Bit Operations/Compare To Constant  relop===  const=3  OutDataTypeStr=boolean
  Compare To Constant3 : simulink/Logic and Bit Operations/Compare To Constant  relop===  const=4  OutDataTypeStr=boolean
  Compare To Constant4 : simulink/Logic and Bit Operations/Compare To Constant  relop===  const=5  OutDataTypeStr=boolean
  Compare To Constant5 : simulink/Logic and Bit Operations/Compare To Constant  relop===  const=6  OutDataTypeStr=boolean
  Compare To Constant6 : simulink/Logic and Bit Operations/Compare To Constant  relop===  const=7  OutDataTypeStr=boolean
  Compare To Constant7 : simulink/Logic and Bit Operations/Compare To Constant  relop===  const=0  OutDataTypeStr=boolean
  Compare To Constant8 : simulink/Logic and Bit Operations/Compare To Constant  relop===  const=8  OutDataTypeStr=boolean
  Compare To Constant9 : simulink/Logic and Bit Operations/Compare To Constant  relop===  const=9  OutDataTypeStr=boolean
  Display : Display
  W0 : Outport
  W1 : Outport  Port=2
  W2 : Outport  Port=3
  W3 : Outport  Port=4
  W4 : Outport  Port=5
  W5 : Outport  Port=6
  W6 : Outport  Port=7
  W7 : Outport  Port=8
  W8 : Outport  Port=9
  W9 : Outport  Port=10
  W10 : Outport  Port=11
  W11 : Outport  Port=12
  W12 : Outport  Port=13
  W13 : Outport  Port=14
  W14 : Outport  Port=15
  W15 : Outport  Port=16
  wires:
  AND/1 -> W0/1
  AND1/1 -> W1/1
  AND3/1 -> Display/1, W3/1
  AND4/1 -> W4/1
  AND5/1 -> W5/1
  AND6/1 -> W6/1
  AND7/1 -> W7/1
  Compare To Constant7/1 -> AND/1
  Compare To Constant/1 -> AND1/1
  Compare To Constant1/1 -> AND2/1
  Compare To Constant4/1 -> AND5/1
  Compare To Constant3/1 -> AND4/1
  Compare To Constant2/1 -> AND3/1
  Compare To Constant6/1 -> AND7/1
  Compare To Constant5/1 -> AND6/1
  AND2/1 -> W2/1
  AND8/1 -> W8/1
  Compare To Constant8/1 -> AND8/1
  Compare To Constant13/1 -> AND13/1
  AND13/1 -> W13/1
  Compare To Constant9/1 -> AND9/1
  Compare To Constant10/1 -> AND10/1
  Compare To Constant11/1 -> AND11/1
  AND12/1 -> W12/1
  AND9/1 -> W9/1
  AND10/1 -> W10/1
  AND11/1 -> W11/1
  Compare To Constant12/1 -> AND12/1
  Compare To Constant15/1 -> AND15/1
  AND14/1 -> W14/1
  WriteAddress/1 -> Compare To Constant15/1, Compare To Constant14/1, Compare To Constant13/1, Compare To Constant12/1, Compare To Constant11/1, Compare To Constant10/1, Compare To Constant9/1, Compare To Constant8/1, Compare To Constant6/1, Compare To Constant5/1, Compare To Constant4/1, Compare To Constant3/1, Compare To Constant2/1, Compare To Constant1/1, Compare To Constant/1, Compare To Constant7/1
  AND15/1 -> W15/1
  Compare To Constant14/1 -> AND14/1
  RegWrite/1 -> AND/2, AND1/2, AND5/2, AND10/2, AND15/2, AND14/2, AND13/2, AND12/2, AND11/2, AND9/2, AND8/2, AND7/2, AND6/2, AND4/2, AND3/2, AND2/2

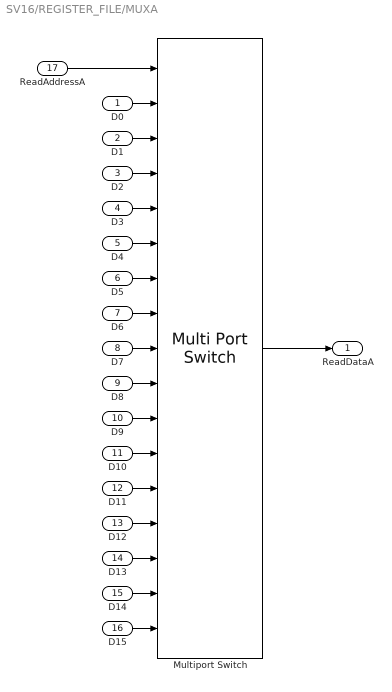
== system SV16/REGISTER_FILE/MUXA ==
  D0 : Inport
  D1 : Inport  Port=2
  D2 : Inport  Port=3
  D3 : Inport  Port=4
  D4 : Inport  Port=5
  D5 : Inport  Port=6
  D6 : Inport  Port=7
  D7 : Inport  Port=8
  D8 : Inport  Port=9
  D9 : Inport  Port=10
  D10 : Inport  Port=11
  D11 : Inport  Port=12
  D12 : Inport  Port=13
  D13 : Inport  Port=14
  D14 : Inport  Port=15
  D15 : Inport  Port=16
  ReadAddressA : Inport  Port=17
  Multiport Switch : MultiPortSwitch  DataPortOrder=Zero-based contiguous  Inputs=16  zeroidx=on  OutDataTypeStr=uint16  SaturateOnIntegerOverflow=off  InputSameDT=off
  ReadDataA : Outport  OutDataTypeStr=uint16
  wires:
  D0/1 -> Multiport Switch/2
  D1/1 -> Multiport Switch/3
  D2/1 -> Multiport Switch/4
  D3/1 -> Multiport Switch/5
  D4/1 -> Multiport Switch/6
  D5/1 -> Multiport Switch/7
  D6/1 -> Multiport Switch/8
  D7/1 -> Multiport Switch/9
  ReadAddressA/1 -> Multiport Switch/1
  Multiport Switch/1 -> ReadDataA/1
  D10/1 -> Multiport Switch/12
  D12/1 -> Multiport Switch/14
  D14/1 -> Multiport Switch/16
  D11/1 -> Multiport Switch/13
  D15/1 -> Multiport Switch/17
  D9/1 -> Multiport Switch/11
  D8/1 -> Multiport Switch/10
  D13/1 -> Multiport Switch/15

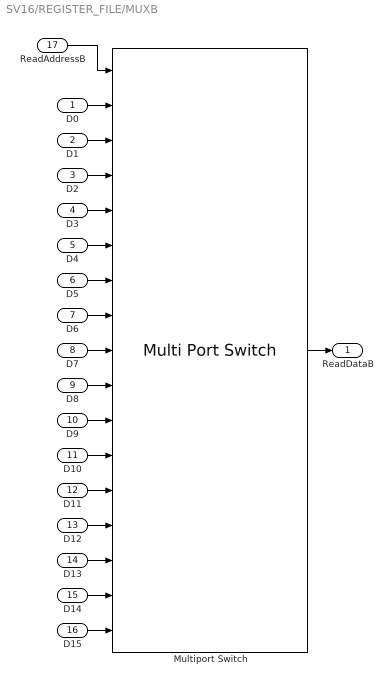
== system SV16/REGISTER_FILE/MUXB ==
  D0 : Inport
  D1 : Inport  Port=2
  D2 : Inport  Port=3
  D3 : Inport  Port=4
  D4 : Inport  Port=5
  D5 : Inport  Port=6
  D6 : Inport  Port=7
  D7 : Inport  Port=8
  D8 : Inport  Port=9
  D9 : Inport  Port=10
  D10 : Inport  Port=11
  D11 : Inport  Port=12
  D12 : Inport  Port=13
  D13 : Inport  Port=14
  D14 : Inport  Port=15
  D15 : Inport  Port=16
  ReadAddressB : Inport  Port=17
  Multiport Switch : MultiPortSwitch  DataPortOrder=Zero-based contiguous  Inputs=16  zeroidx=on  OutDataTypeStr=uint16  SaturateOnIntegerOverflow=off  InputSameDT=off
  ReadDataB : Outport  OutDataTypeStr=uint16
  wires:
  D0/1 -> Multiport Switch/2
  D1/1 -> Multiport Switch/3
  D2/1 -> Multiport Switch/4
  D3/1 -> Multiport Switch/5
  D4/1 -> Multiport Switch/6
  D5/1 -> Multiport Switch/7
  D6/1 -> Multiport Switch/8
  D7/1 -> Multiport Switch/9
  ReadAddressB/1 -> Multiport Switch/1
  Multiport Switch/1 -> ReadDataB/1
  D10/1 -> Multiport Switch/12
  D12/1 -> Multiport Switch/14
  D14/1 -> Multiport Switch/16
  D11/1 -> Multiport Switch/13
  D15/1 -> Multiport Switch/17
  D9/1 -> Multiport Switch/11
  D8/1 -> Multiport Switch/10
  D13/1 -> Multiport Switch/15

== system SV16/REGISTER_FILE/R0 ==
  D : Inport
  WE : Inport  Port=2
  Reset : Inport  Port=3
  Constant : Constant  Value=0  OutDataTypeStr=uint16
  Constant1 : Constant  OutDataTypeStr=uint16
  Switch : Switch  Criteria=u2 > Threshold  SaturateOnIntegerOverflow=off  InputSameDT=off
  Switch1 : Switch  Criteria=u2 > Threshold  SaturateOnIntegerOverflow=off  InputSameDT=off
  Unit Delay Enabled Synchronous : hdlsllib/Discrete/Unit Delay Enabled Synchronous  InitialCondition=0.0  SampleTime=-1
  D0 : Outport
  wires:
  D/1 -> Switch/1
  WE/1 -> Switch/2
  Unit Delay Enabled Synchronous/1 -> D0/1, Switch/3
  Reset/1 -> Switch1/2
  Constant/1 -> Switch1/1
  Switch/1 -> Switch1/3
  Switch1/1 -> Unit Delay Enabled Synchronous/1
  Constant1/1 -> Unit Delay Enabled Synchronous/2

== system SV16/REGISTER_FILE/R1 ==
  D : Inport
  WE : Inport  Port=2
  Reset : Inport  Port=3
  Constant : Constant  Value=0  OutDataTypeStr=uint16
  Constant1 : Constant  OutDataTypeStr=uint16
  Switch : Switch  Criteria=u2 > Threshold  SaturateOnIntegerOverflow=off  InputSameDT=off
  Switch1 : Switch  Criteria=u2 > Threshold  SaturateOnIntegerOverflow=off  InputSameDT=off
  Unit Delay Enabled Synchronous : hdlsllib/Discrete/Unit Delay Enabled Synchronous  InitialCondition=0.0  SampleTime=-1
  D1 : Outport
  wires:
  D/1 -> Switch/1
  WE/1 -> Switch/2
  Unit Delay Enabled Synchronous/1 -> D1/1, Switch/3
  Reset/1 -> Switch1/2
  Constant/1 -> Switch1/1
  Switch/1 -> Switch1/3
  Switch1/1 -> Unit Delay Enabled Synchronous/1
  Constant1/1 -> Unit Delay Enabled Synchronous/2

== system SV16/REGISTER_FILE/R10 ==
  D : Inport
  WE : Inport  Port=2
  Reset : Inport  Port=3
  Constant : Constant  Value=0  OutDataTypeStr=uint16
  Constant1 : Constant  OutDataTypeStr=uint16
  Switch : Switch  Criteria=u2 > Threshold  SaturateOnIntegerOverflow=off  InputSameDT=off
  Switch1 : Switch  Criteria=u2 > Threshold  SaturateOnIntegerOverflow=off  InputSameDT=off
  Unit Delay Enabled Synchronous : hdlsllib/Discrete/Unit Delay Enabled Synchronous  InitialCondition=0.0  SampleTime=-1
  D10 : Outport
  wires:
  D/1 -> Switch/1
  WE/1 -> Switch/2
  Unit Delay Enabled Synchronous/1 -> D10/1, Switch/3
  Reset/1 -> Switch1/2
  Constant/1 -> Switch1/1
  Switch/1 -> Switch1/3
  Switch1/1 -> Unit Delay Enabled Synchronous/1
  Constant1/1 -> Unit Delay Enabled Synchronous/2

== system SV16/REGISTER_FILE/R11 ==
  D : Inport
  WE : Inport  Port=2
  Reset : Inport  Port=3
  Constant : Constant  Value=0  OutDataTypeStr=uint16
  Constant1 : Constant  OutDataTypeStr=uint16
  Switch : Switch  Criteria=u2 > Threshold  SaturateOnIntegerOverflow=off  InputSameDT=off
  Switch1 : Switch  Criteria=u2 > Threshold  SaturateOnIntegerOverflow=off  InputSameDT=off
  Unit Delay Enabled Synchronous : hdlsllib/Discrete/Unit Delay Enabled Synchronous  InitialCondition=0.0  SampleTime=-1
  D11 : Outport
  wires:
  D/1 -> Switch/1
  WE/1 -> Switch/2
  Unit Delay Enabled Synchronous/1 -> D11/1, Switch/3
  Reset/1 -> Switch1/2
  Constant/1 -> Switch1/1
  Switch/1 -> Switch1/3
  Switch1/1 -> Unit Delay Enabled Synchronous/1
  Constant1/1 -> Unit Delay Enabled Synchronous/2

== system SV16/REGISTER_FILE/R12 ==
  D : Inport
  WE : Inport  Port=2
  Reset : Inport  Port=3
  Constant : Constant  Value=0  OutDataTypeStr=uint16
  Constant1 : Constant  OutDataTypeStr=uint16
  Switch : Switch  Criteria=u2 > Threshold  SaturateOnIntegerOverflow=off  InputSameDT=off
  Switch1 : Switch  Criteria=u2 > Threshold  SaturateOnIntegerOverflow=off  InputSameDT=off
  Unit Delay Enabled Synchronous : hdlsllib/Discrete/Unit Delay Enabled Synchronous  InitialCondition=0.0  SampleTime=-1
  D12 : Outport
  wires:
  D/1 -> Switch/1
  WE/1 -> Switch/2
  Unit Delay Enabled Synchronous/1 -> D12/1, Switch/3
  Reset/1 -> Switch1/2
  Constant/1 -> Switch1/1
  Switch/1 -> Switch1/3
  Switch1/1 -> Unit Delay Enabled Synchronous/1
  Constant1/1 -> Unit Delay Enabled Synchronous/2

== system SV16/REGISTER_FILE/R13 ==
  D : Inport
  WE : Inport  Port=2
  Reset : Inport  Port=3
  Constant : Constant  Value=0  OutDataTypeStr=uint16
  Constant1 : Constant  OutDataTypeStr=uint16
  Switch : Switch  Criteria=u2 > Threshold  SaturateOnIntegerOverflow=off  InputSameDT=off
  Switch1 : Switch  Criteria=u2 > Threshold  SaturateOnIntegerOverflow=off  InputSameDT=off
  Unit Delay Enabled Synchronous : hdlsllib/Discrete/Unit Delay Enabled Synchronous  InitialCondition=0.0  SampleTime=-1
  D13 : Outport
  wires:
  D/1 -> Switch/1
  WE/1 -> Switch/2
  Unit Delay Enabled Synchronous/1 -> D13/1, Switch/3
  Reset/1 -> Switch1/2
  Constant/1 -> Switch1/1
  Switch/1 -> Switch1/3
  Switch1/1 -> Unit Delay Enabled Synchronous/1
  Constant1/1 -> Unit Delay Enabled Synchronous/2

== system SV16/REGISTER_FILE/R14 ==
  D : Inport
  WE : Inport  Port=2
  Reset : Inport  Port=3
  Constant : Constant  Value=0  OutDataTypeStr=uint16
  Constant1 : Constant  OutDataTypeStr=uint16
  Switch : Switch  Criteria=u2 > Threshold  SaturateOnIntegerOverflow=off  InputSameDT=off
  Switch1 : Switch  Criteria=u2 > Threshold  SaturateOnIntegerOverflow=off  InputSameDT=off
  Unit Delay Enabled Synchronous : hdlsllib/Discrete/Unit Delay Enabled Synchronous  InitialCondition=0.0  SampleTime=-1
  D14 : Outport
  wires:
  D/1 -> Switch/1
  WE/1 -> Switch/2
  Unit Delay Enabled Synchronous/1 -> D14/1, Switch/3
  Reset/1 -> Switch1/2
  Constant/1 -> Switch1/1
  Switch/1 -> Switch1/3
  Switch1/1 -> Unit Delay Enabled Synchronous/1
  Constant1/1 -> Unit Delay Enabled Synchronous/2

== system SV16/REGISTER_FILE/R15 ==
  D : Inport
  WE : Inport  Port=2
  Reset : Inport  Port=3
  Constant : Constant  Value=0  OutDataTypeStr=uint16
  Constant1 : Constant  OutDataTypeStr=uint16
  Switch : Switch  Criteria=u2 > Threshold  SaturateOnIntegerOverflow=off  InputSameDT=off
  Switch1 : Switch  Criteria=u2 > Threshold  SaturateOnIntegerOverflow=off  InputSameDT=off
  Unit Delay Enabled Synchronous : hdlsllib/Discrete/Unit Delay Enabled Synchronous  InitialCondition=0.0  SampleTime=-1
  D15 : Outport
  wires:
  D/1 -> Switch/1
  WE/1 -> Switch/2
  Unit Delay Enabled Synchronous/1 -> D15/1, Switch/3
  Reset/1 -> Switch1/2
  Constant/1 -> Switch1/1
  Switch/1 -> Switch1/3
  Switch1/1 -> Unit Delay Enabled Synchronous/1
  Constant1/1 -> Unit Delay Enabled Synchronous/2

== system SV16/REGISTER_FILE/R2 ==
  D : Inport
  WE : Inport  Port=2
  Reset : Inport  Port=3
  Constant : Constant  Value=0  OutDataTypeStr=uint16
  Constant1 : Constant  OutDataTypeStr=uint16
  Switch : Switch  Criteria=u2 > Threshold  SaturateOnIntegerOverflow=off  InputSameDT=off
  Switch1 : Switch  Criteria=u2 > Threshold  SaturateOnIntegerOverflow=off  InputSameDT=off
  Unit Delay Enabled Synchronous : hdlsllib/Discrete/Unit Delay Enabled Synchronous  InitialCondition=0.0  SampleTime=-1
  D2 : Outport
  wires:
  D/1 -> Switch/1
  WE/1 -> Switch/2
  Unit Delay Enabled Synchronous/1 -> D2/1, Switch/3
  Reset/1 -> Switch1/2
  Constant/1 -> Switch1/1
  Switch/1 -> Switch1/3
  Switch1/1 -> Unit Delay Enabled Synchronous/1
  Constant1/1 -> Unit Delay Enabled Synchronous/2

== system SV16/REGISTER_FILE/R3 ==
  D : Inport
  WE : Inport  Port=2
  Reset : Inport  Port=3
  Constant : Constant  Value=0  OutDataTypeStr=uint16
  Constant1 : Constant  OutDataTypeStr=uint16
  Switch : Switch  Criteria=u2 > Threshold  SaturateOnIntegerOverflow=off  InputSameDT=off
  Switch1 : Switch  Criteria=u2 > Threshold  SaturateOnIntegerOverflow=off  InputSameDT=off
  Unit Delay Enabled Synchronous : hdlsllib/Discrete/Unit Delay Enabled Synchronous  InitialCondition=0.0  SampleTime=-1
  D3 : Outport
  wires:
  D/1 -> Switch/1
  WE/1 -> Switch/2
  Unit Delay Enabled Synchronous/1 -> D3/1, Switch/3
  Reset/1 -> Switch1/2
  Constant/1 -> Switch1/1
  Switch/1 -> Switch1/3
  Switch1/1 -> Unit Delay Enabled Synchronous/1
  Constant1/1 -> Unit Delay Enabled Synchronous/2

== system SV16/REGISTER_FILE/R4 ==
  D : Inport
  WE : Inport  Port=2
  Reset : Inport  Port=3
  Constant : Constant  Value=0  OutDataTypeStr=uint16
  Constant1 : Constant  OutDataTypeStr=uint16
  Switch : Switch  Criteria=u2 > Threshold  SaturateOnIntegerOverflow=off  InputSameDT=off
  Switch1 : Switch  Criteria=u2 > Threshold  SaturateOnIntegerOverflow=off  InputSameDT=off
  Unit Delay Enabled Synchronous : hdlsllib/Discrete/Unit Delay Enabled Synchronous  InitialCondition=0.0  SampleTime=-1
  D4 : Outport
  wires:
  D/1 -> Switch/1
  WE/1 -> Switch/2
  Unit Delay Enabled Synchronous/1 -> D4/1, Switch/3
  Reset/1 -> Switch1/2
  Constant/1 -> Switch1/1
  Switch/1 -> Switch1/3
  Switch1/1 -> Unit Delay Enabled Synchronous/1
  Constant1/1 -> Unit Delay Enabled Synchronous/2

== system SV16/REGISTER_FILE/R5 ==
  D : Inport
  WE : Inport  Port=2
  Reset : Inport  Port=3
  Constant : Constant  Value=0  OutDataTypeStr=uint16
  Constant1 : Constant  OutDataTypeStr=uint16
  Switch : Switch  Criteria=u2 > Threshold  SaturateOnIntegerOverflow=off  InputSameDT=off
  Switch1 : Switch  Criteria=u2 > Threshold  SaturateOnIntegerOverflow=off  InputSameDT=off
  Unit Delay Enabled Synchronous : hdlsllib/Discrete/Unit Delay Enabled Synchronous  InitialCondition=0.0  SampleTime=-1
  D5 : Outport
  wires:
  D/1 -> Switch/1
  WE/1 -> Switch/2
  Unit Delay Enabled Synchronous/1 -> D5/1, Switch/3
  Reset/1 -> Switch1/2
  Constant/1 -> Switch1/1
  Switch/1 -> Switch1/3
  Switch1/1 -> Unit Delay Enabled Synchronous/1
  Constant1/1 -> Unit Delay Enabled Synchronous/2

== system SV16/REGISTER_FILE/R6 ==
  D : Inport
  WE : Inport  Port=2
  Reset : Inport  Port=3
  Constant : Constant  Value=0  OutDataTypeStr=uint16
  Constant1 : Constant  OutDataTypeStr=uint16
  Switch : Switch  Criteria=u2 > Threshold  SaturateOnIntegerOverflow=off  InputSameDT=off
  Switch1 : Switch  Criteria=u2 > Threshold  SaturateOnIntegerOverflow=off  InputSameDT=off
  Unit Delay Enabled Synchronous : hdlsllib/Discrete/Unit Delay Enabled Synchronous  InitialCondition=0.0  SampleTime=-1
  D6 : Outport
  wires:
  D/1 -> Switch/1
  WE/1 -> Switch/2
  Unit Delay Enabled Synchronous/1 -> D6/1, Switch/3
  Reset/1 -> Switch1/2
  Constant/1 -> Switch1/1
  Switch/1 -> Switch1/3
  Switch1/1 -> Unit Delay Enabled Synchronous/1
  Constant1/1 -> Unit Delay Enabled Synchronous/2

== system SV16/REGISTER_FILE/R7 ==
  D : Inport
  WE : Inport  Port=2
  Reset : Inport  Port=3
  Constant : Constant  Value=0  OutDataTypeStr=uint16
  Constant1 : Constant  OutDataTypeStr=uint16
  Switch : Switch  Criteria=u2 > Threshold  SaturateOnIntegerOverflow=off  InputSameDT=off
  Switch1 : Switch  Criteria=u2 > Threshold  SaturateOnIntegerOverflow=off  InputSameDT=off
  Unit Delay Enabled Synchronous : hdlsllib/Discrete/Unit Delay Enabled Synchronous  InitialCondition=0.0  SampleTime=-1
  D7 : Outport
  wires:
  D/1 -> Switch/1
  WE/1 -> Switch/2
  Unit Delay Enabled Synchronous/1 -> D7/1, Switch/3
  Reset/1 -> Switch1/2
  Constant/1 -> Switch1/1
  Switch/1 -> Switch1/3
  Switch1/1 -> Unit Delay Enabled Synchronous/1
  Constant1/1 -> Unit Delay Enabled Synchronous/2

== system SV16/REGISTER_FILE/R8 ==
  D : Inport
  WE : Inport  Port=2
  Reset : Inport  Port=3
  Constant : Constant  Value=0  OutDataTypeStr=uint16
  Constant1 : Constant  OutDataTypeStr=uint16
  Switch : Switch  Criteria=u2 > Threshold  SaturateOnIntegerOverflow=off  InputSameDT=off
  Switch1 : Switch  Criteria=u2 > Threshold  SaturateOnIntegerOverflow=off  InputSameDT=off
  Unit Delay Enabled Synchronous : hdlsllib/Discrete/Unit Delay Enabled Synchronous  InitialCondition=0.0  SampleTime=-1
  D8 : Outport
  wires:
  D/1 -> Switch/1
  WE/1 -> Switch/2
  Unit Delay Enabled Synchronous/1 -> D8/1, Switch/3
  Reset/1 -> Switch1/2
  Constant/1 -> Switch1/1
  Switch/1 -> Switch1/3
  Switch1/1 -> Unit Delay Enabled Synchronous/1
  Constant1/1 -> Unit Delay Enabled Synchronous/2

== system SV16/REGISTER_FILE/R9 ==
  D : Inport
  WE : Inport  Port=2
  Reset : Inport  Port=3
  Constant : Constant  Value=0  OutDataTypeStr=uint16
  Constant1 : Constant  OutDataTypeStr=uint16
  Switch : Switch  Criteria=u2 > Threshold  SaturateOnIntegerOverflow=off  InputSameDT=off
  Switch1 : Switch  Criteria=u2 > Threshold  SaturateOnIntegerOverflow=off  InputSameDT=off
  Unit Delay Enabled Synchronous : hdlsllib/Discrete/Unit Delay Enabled Synchronous  InitialCondition=0.0  SampleTime=-1
  D9 : Outport
  wires:
  D/1 -> Switch/1
  WE/1 -> Switch/2
  Unit Delay Enabled Synchronous/1 -> D9/1, Switch/3
  Reset/1 -> Switch1/2
  Constant/1 -> Switch1/1
  Switch/1 -> Switch1/3
  Switch1/1 -> Unit Delay Enabled Synchronous/1
  Constant1/1 -> Unit Delay Enabled Synchronous/2

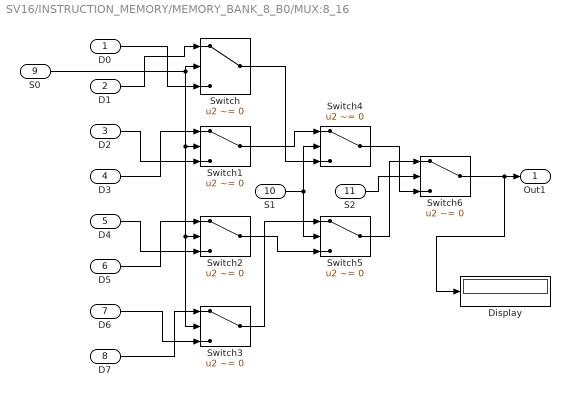
== system SV16/INSTRUCTION_MEMORY/MEMORY_BANK_8_B0/MUX:8_16 ==
  D0 : Inport  OutDataTypeStr=uint32
  D1 : Inport  Port=2  OutDataTypeStr=uint32
  D2 : Inport  Port=3  OutDataTypeStr=uint32
  D3 : Inport  Port=4  OutDataTypeStr=uint32
  D4 : Inport  Port=5  OutDataTypeStr=uint32
  D5 : Inport  Port=6  OutDataTypeStr=uint32
  D6 : Inport  Port=7  OutDataTypeStr=uint32
  D7 : Inport  Port=8  OutDataTypeStr=uint32
  S0 : Inport  Port=9  OutDataTypeStr=boolean
  S1 : Inport  Port=10  OutDataTypeStr=boolean
  S2 : Inport  Port=11  OutDataTypeStr=boolean
  Display : Display
  Switch{,1..6} (7 alike) : Switch  Criteria=u2 ~= 0  SaturateOnIntegerOverflow=off  InputSameDT=off
  Out1 : Outport  OutDataTypeStr=uint32
  wires:
  D0/1 -> Switch/3
  S0/1 -> Switch/2, Switch3/2, Switch2/2, Switch1/2
  D3/1 -> Switch1/1
  D5/1 -> Switch2/1
  D6/1 -> Switch3/3
  Switch/1 -> Switch4/3
  S1/1 -> Switch5/2, Switch4/2
  S2/1 -> Switch6/2
  Switch6/1 -> Display/1, Out1/1
  D1/1 -> Switch/1
  D2/1 -> Switch1/3
  D4/1 -> Switch2/3
  D7/1 -> Switch3/1
  Switch4/1 -> Switch6/3
  Switch5/1 -> Switch6/1
  Switch1/1 -> Switch4/1
  Switch2/1 -> Switch5/3
  Switch3/1 -> Switch5/1

== system SV16/INSTRUCTION_MEMORY/MEMORY_BANK_8_B0/R0 ==
  D : Inport
  WE : Inport  Port=2
  Reset : Inport  Port=3
  Constant : Constant  Value=0  OutDataTypeStr=uint16
  Constant1 : Constant  OutDataTypeStr=uint32
  Subsystem : Subsystem
  Switch : Switch  Criteria=u2 > Threshold  SaturateOnIntegerOverflow=off  InputSameDT=off
  Switch1 : Switch  Criteria=u2 > Threshold  SaturateOnIntegerOverflow=off  InputSameDT=off
  D0 : Outport  OutDataTypeStr=uint32
  wires:
  D/1 -> Switch/1
  WE/1 -> Switch/2
  Reset/1 -> Switch1/2
  Constant/1 -> Switch1/1
  Switch/1 -> Switch1/3
  Subsystem/1(y) -> D0/1, Switch/3
  Switch1/1 -> Subsystem/1(u)
  Constant1/1 -> Subsystem/2(E)

== system SV16/INSTRUCTION_MEMORY/MEMORY_BANK_8_B0/R1 ==
  D : Inport
  WE : Inport  Port=2
  Reset : Inport  Port=3
  Constant : Constant  Value=0  OutDataTypeStr=uint16
  Constant1 : Constant  OutDataTypeStr=uint16
  Switch : Switch  Criteria=u2 > Threshold  SaturateOnIntegerOverflow=off  InputSameDT=off
  Switch1 : Switch  Criteria=u2 > Threshold  SaturateOnIntegerOverflow=off  InputSameDT=off
  Unit Delay Enabled Synchronous : hdlsllib/Discrete/Unit Delay Enabled Synchronous  InitialCondition=0.0  SampleTime=-1
  D1 : Outport
  wires:
  D/1 -> Switch/1
  WE/1 -> Switch/2
  Unit Delay Enabled Synchronous/1 -> D1/1, Switch/3
  Reset/1 -> Switch1/2
  Constant/1 -> Switch1/1
  Switch/1 -> Switch1/3
  Switch1/1 -> Unit Delay Enabled Synchronous/1
  Constant1/1 -> Unit Delay Enabled Synchronous/2

== system SV16/INSTRUCTION_MEMORY/MEMORY_BANK_8_B0/R2 ==
  D : Inport
  WE : Inport  Port=2
  Reset : Inport  Port=3
  Constant : Constant  Value=0  OutDataTypeStr=uint16
  Constant1 : Constant  OutDataTypeStr=uint16
  Switch : Switch  Criteria=u2 > Threshold  SaturateOnIntegerOverflow=off  InputSameDT=off
  Switch1 : Switch  Criteria=u2 > Threshold  SaturateOnIntegerOverflow=off  InputSameDT=off
  Unit Delay Enabled Synchronous : hdlsllib/Discrete/Unit Delay Enabled Synchronous  InitialCondition=0.0  SampleTime=-1
  D2 : Outport
  wires:
  D/1 -> Switch/1
  WE/1 -> Switch/2
  Unit Delay Enabled Synchronous/1 -> D2/1, Switch/3
  Reset/1 -> Switch1/2
  Constant/1 -> Switch1/1
  Switch/1 -> Switch1/3
  Switch1/1 -> Unit Delay Enabled Synchronous/1
  Constant1/1 -> Unit Delay Enabled Synchronous/2

== system SV16/INSTRUCTION_MEMORY/MEMORY_BANK_8_B0/R3 ==
  D : Inport
  WE : Inport  Port=2
  Reset : Inport  Port=3
  Constant : Constant  Value=0  OutDataTypeStr=uint16
  Constant1 : Constant  OutDataTypeStr=uint16
  Switch : Switch  Criteria=u2 > Threshold  SaturateOnIntegerOverflow=off  InputSameDT=off
  Switch1 : Switch  Criteria=u2 > Threshold  SaturateOnIntegerOverflow=off  InputSameDT=off
  Unit Delay Enabled Synchronous : hdlsllib/Discrete/Unit Delay Enabled Synchronous  InitialCondition=0.0  SampleTime=-1
  D3 : Outport
  wires:
  D/1 -> Switch/1
  WE/1 -> Switch/2
  Unit Delay Enabled Synchronous/1 -> D3/1, Switch/3
  Reset/1 -> Switch1/2
  Constant/1 -> Switch1/1
  Switch/1 -> Switch1/3
  Switch1/1 -> Unit Delay Enabled Synchronous/1
  Constant1/1 -> Unit Delay Enabled Synchronous/2
